simulink model "Math"  (R2020a)
settings: Solver=FixedStepDiscrete  StartTime=0.0  StopTime=10.0  RelTol=1e-3
libraries: simulink x1
settings Model: Creator=sadamu  LastModifiedBy=sadamu
settings OptimizationCC: OptimizeBlockIOStorage=off  OptimizeDataStoreBuffers=off  BusAssignmentInplaceUpdate=off
settings DebuggingCC: SFUnexpectedBacktrackingDiag=warning  SFNoUnconditionalDefaultTransitionDiag=warning
settings RTWCC: GenerateReport=on  BuildConfiguration=Debug  LaunchReport=on
settings CodeAppCC: GenerateComments=off  MATLABSourceComments=on  EnableCustomComments=on
settings GRTTargetCC: CombineSignalStateStructs=on  SupportVariableSizeSignals=on  MultiInstanceErrorCode=Warning

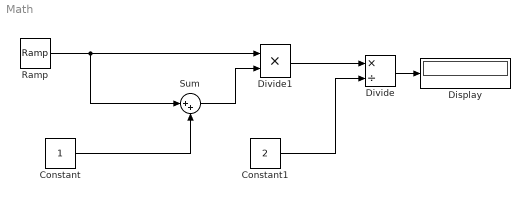
== system Math ==
  Constant : Constant
  Constant1 : Constant  Value=2
  Display : Display
  Divide : Product  Inputs=*/
  Divide1 : Product  Inputs=**
  Ramp : simulink/Sources/Ramp  slope=1  start=0  InitialOutput=0
  Sum : Sum  Inputs=|++
  wires:
  Divide/1 -> Display/1
  Ramp/1 -> Divide1/1, Sum/1
  Constant/1 -> Sum/2
  Constant1/1 -> Divide/2
  Divide1/1 -> Divide/1
  Sum/1 -> Divide1/2
